simulink model "nav"  (R2025b)
settings: Solver=ode2  StartTime=0.0  StopTime=inf  FixedStep=1/100  RelTol=1e-3
PreLoadFcn:
  | nav_PreLoadFcn
  | stepsize_ctrl = evalin('base', get_param(bdroot, 'FixedStep'));
values from neighbouring files (symbols this model uses):
  navConsts = defineConstants_nav()    [nav_PreLoadFcn.m]
undefined symbols (not defined in the file or in its folder): dspblkCoreblockFVToolHelper, gcbh
libraries: eeGeneralControl x5, simulink x2, sharedutil x1, sharedtransform x1
(part 1 of 2)
settings Model: Creator=ac112430  LastModifiedBy=ac124458
settings SolverCC: AlgebraicLoopSolver=TrustRegion
settings DataIOCC: ReturnWorkspaceOutputs=off
settings OptimizationCC: DefaultParameterBehavior=Inlined  DefaultUnderspecifiedDataType=single  PassReuseOutputArgsAs=Individual arguments  EfficientTunableParamExpr=on
settings DebuggingCC: ParameterPrecisionLossMsg=none  ParameterTunabilityLossMsg=error  UnconnectedInputMsg=warning  UnconnectedOutputMsg=warning  UnconnectedLineMsg=warning  BusObjectLabelMismatch=none  ArithmeticOperatorsInVariantConditions=warning
settings HardwareCC: ProdBitPerPointer=32.0  ProdBitPerSizeT=32.0  ProdBitPerPtrDiffT=32.0  ProdLargestAtomicInteger=Long  ProdLargestAtomicFloat=Double  ProdIntDivRoundTo=Undefined  ProdWordSize=32.0  ProdHWDeviceType=ARM Compatible->ARM Cortex
settings ModelReferenceCC: EnableRefExpFcnMdlSchedulingChecks=on  ModelReferenceNumInstancesAllowed=Single  PropagateSignalLabelsOutOfModel=off
settings SFSimCC: SimUseLocalCustomCode=off  MATLABDynamicMemAlloc=off  CustomCodeUndefinedFunction=UseInterfaceOnly
settings RTWCC: SystemTargetFile=ert.tlc  GenCodeOnly=on  TemplateMakefile=ert_default_tmf  RTWUseLocalCustomCode=off  IncludeHyperlinkInReport=on  GPUComputeCapability=3.5  Description=Embedded Coder
settings CodeAppCC: IgnoreCustomStorageClasses=off  MaxIdLength=2048.0  StateflowObjectComments=on
settings ERTTargetCC: ERTCustomFileTemplate=example_file_process.tlc  ConvertIfToSwitch=off  SuppressUnreachableDefaultCases=off  DynamicArrayContainerType=coder::array  TargetLangStandard=C99 (ISO)  GenerateSampleERTMain=on  SubcomponentCodeInterfacePackaging=Nonreusable function  SupportNonFinite=off  SupportComplex=off

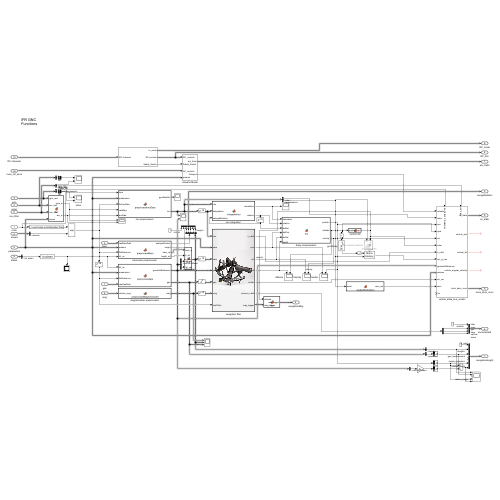
[thumbnail: Simulink's stored preview of the top-level diagram]
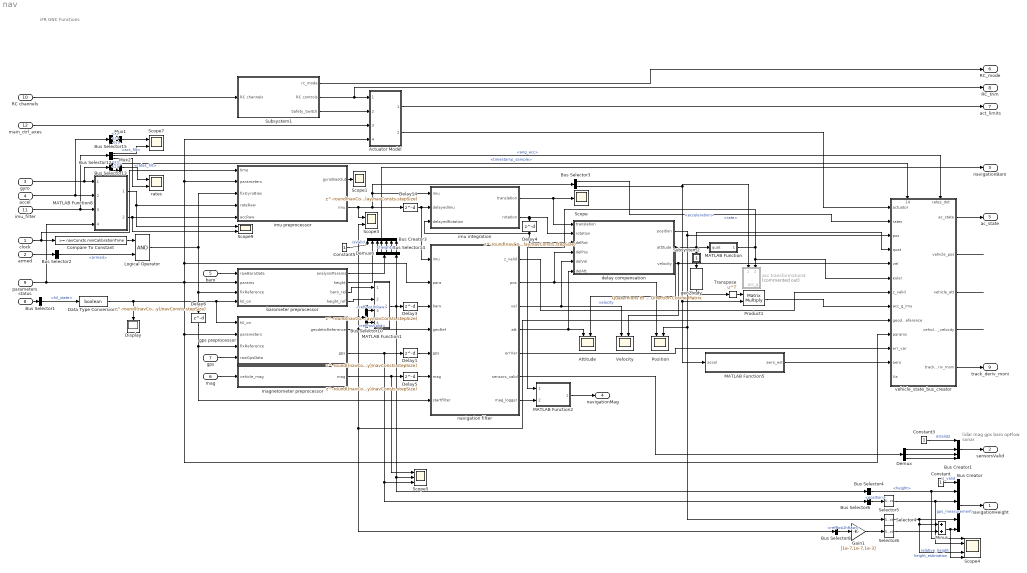
== system nav ==
  note: lidar
      | mag
      | gps
      | baro
      | opFlow
      | sonar
  note: iFR GNC Functions
  clock : Inport  OutDataTypeStr=single
  armed : Inport  Port=2  OutDataTypeStr=Bus: actuator_armed_bus
  gyro : Inport  Port=3  OutDataTypeStr=Bus: sensor_gyro_bus
  accel : Inport  Port=4  OutDataTypeStr=Bus: sensor_accel_bus
  baro : Inport  Port=5  OutDataTypeStr=Bus: sensor_baro_bus
  mag : Inport  Port=6  OutDataTypeStr=Bus: vehicle_magnetometer_bus
  gps : Inport  Port=7  OutDataTypeStr=Bus: vehicle_gps_position_bus
  status : Inport  Port=8  OutDataTypeStr=Bus: vehicle_status_bus  Interpolate=off  BusOutputAsStruct=on
  parameters : Inport  Port=9  OutDataTypeStr=Bus: nav_parameterBus
  RC channels : Inport  Port=10  OutDataTypeStr=Bus: rc_channels_bus
  imu_filter : Inport  Port=11  OutDataTypeStr=Bus: ifr_imu_filtered_bus
  main_ctrl_axes : Inport  Port=12  OutDataTypeStr=Bus: main_ctrl_axes_bus
  Actuator Model : Subsystem
  Attitude : Scope  NumInputPorts=2
      settings: ActiveDisplayYMinimum=-1.23773  ActiveDisplayYMaximum=1.24864
  Bus Creator : BusCreator  Inputs=6
  Bus Creator1 : BusCreator  Inputs=5
  Bus Creator3 : BusCreator  Inputs=7
  Bus Selector1 : BusSelector  OutputSignals=hil_state
  Bus Selector10 : BusSelector  OutputSignals=refPosLlhRaw,refPosValid
  Bus Selector12 : BusSelector  OutputSignals=acc_filt,ang_acc,rates_filt
  Bus Selector13 : BusSelector  OutputSignals=timestamp_sample,x,y,z
  Bus Selector14 : BusSelector  OutputSignals=height
  Bus Selector15 : BusSelector  OutputSignals=x,y,z
  Bus Selector2 : BusSelector  OutputSignals=armed
  Bus Selector3 : BusSelector  OutputSignals=rate,acceleration
  Bus Selector4 : BusSelector  OutputSignals=height
  Bus Selector6 : BusSelector  OutputSignals=position
  Bus Selector8 : BusSelector  OutputSignals=refPosLlhRaw
  Compare To Constant : simulink/Logic and Bit Operations/Compare To Constant  relop=>=  const=navConsts.minCalibrationTime  OutDataTypeStr=boolean
  Constant : Constant  OutDataTypeStr=boolean
  Constant3 : Constant  OutDataTypeStr=boolean
  Constant5 : Constant  OutDataTypeStr=boolean
  Data Type Conversion1 : DataTypeConversion  OutDataTypeStr=boolean  SaturateOnIntegerOverflow=off  RndMeth=Floor
  Delay1 : Delay  DelayLength=round((navConsts.filterDelay-navConsts.gpsDelay)/navConsts.stepSize)  DelayLengthUpperLimit=300
  Delay14 : Delay  DelayLength=round(navConsts.filterDelay/navConsts.stepSize)  DelayLengthUpperLimit=300
  Delay3 : Delay  DelayLength=round(navConsts.filterDelay/navConsts.stepSize)  DelayLengthUpperLimit=300
  Delay4 : Delay  DelayLength=round(navConsts.filterDelay/navConsts.stepSize)  DelayLengthUpperLimit=300
  Delay5 : Delay  DelayLength=round((navConsts.filterDelay-navConsts.magDelay)/navConsts.stepSize)  DelayLengthUpperLimit=300
  Delay6 : Delay  DelayLength=round((navConsts.filterDelay-navConsts.magDelay)/navConsts.stepSize)  DelayLengthUpperLimit=300
  Demux : Demux  Outputs=3
  Demux6 : Demux
  Display : Display
  Gain1 : Gain  Gain=[1e-7,1e-7,1e-3]  OutDataTypeStr=single
  Logical Operator : Logic  AllPortsSameDT=off  OutDataTypeStr=boolean
  MATLAB Function : MATLAB Function  TreatAsAtomicUnit=on
  MATLAB Function1 : MATLAB Function  TreatAsAtomicUnit=on
  MATLAB Function2 : MATLAB Function  TreatAsAtomicUnit=on
  MATLAB Function5 : MATLAB Function  TreatAsAtomicUnit=on
  MATLAB Function8 : MATLAB Function  TreatAsAtomicUnit=on
  Minus : Sum  OutDataTypeStr=single
  Mux1 : Mux  Inputs=3
  Mux2 : Mux  Inputs=3
  Position : Scope  NumInputPorts=2
      settings: ActiveDisplayYMinimum=-398.4041  ActiveDisplayYMaximum=44.26944  DataLoggingVariableName=ScopeData2
  Product1 : Product  Multiplication=Matrix(*)
  Scope : Scope
      settings: ActiveDisplayYMinimum=-1  ActiveDisplayYMaximum=1  DataLoggingVariableName=ScopeData5
  Scope1 : Scope
      settings: ActiveDisplayYMinimum=-0.099331239782016356  ActiveDisplayYMaximum=0.30195901907356948  DataLoggingVariableName=ScopeData4
  Scope3 : Scope  NumInputPorts=2
      settings: ActiveDisplayYMinimum=-0.2713911799557156  ActiveDisplayYMaximum=0.36740796754492377
  Scope4 : Scope  NumInputPorts=5
      settings: ActiveDisplayYMinimum=349.247314453125  ActiveDisplayYMaximum=356.774169921875
  Scope5 : Scope  NumInputPorts=3
      settings: ActiveDisplayYMinimum=349.247314453125  ActiveDisplayYMaximum=356.774169921875  DataLoggingVariableName=ScopeData2
  Scope7 : Scope  NumInputPorts=2
      settings: ActiveDisplayYMinimum=-34.351112127304077  ActiveDisplayYMaximum=34.884191274642944  DataLoggingVariableName=ScopeData10
  Scope9 : Scope  NumInputPorts=2
      settings: ActiveDisplayYMinimum=-1.8034829497337341  ActiveDisplayYMaximum=1.8379871249198914  DataLoggingVariableName=ScopeData13
  Selector4 : Selector  InputPortWidth=3  IndexOptions=Index vector (dialog)  Indices=[3]  OutputSizes=1
  Selector5 : Selector  InputPortWidth=3  IndexOptions=Index vector (dialog)  Indices=[3]  OutputSizes=1
  Selector6 : Selector  InputPortWidth=3  IndexOptions=Index vector (dialog)  Indices=[3]  OutputSizes=1
  Subsystem1 : Subsystem
  Subsystem2 : Subsystem
  Transpose : Math  Operator=transpose  SignedPower=on
  Velocity : Scope  NumInputPorts=2
      settings: ActiveDisplayYMinimum=-1  ActiveDisplayYMaximum=1  DataLoggingVariableName=ScopeData6
  acc transformation4 : MATLAB Function  Commented=on  TreatAsAtomicUnit=on
  barometer preprocessor : MATLAB Function  TreatAsAtomicUnit=on
  delay compensation : MATLAB Function  TreatAsAtomicUnit=on
  geo2body : sharedtransform/Quaternions to  Direction Cosine Matrix  aMode=aMode
  gps preprocessor : MATLAB Function  TreatAsAtomicUnit=on
  imu integration : MATLAB Function  TreatAsAtomicUnit=on
  imu preprocessor : MATLAB Function  TreatAsAtomicUnit=on
  magnetometer preprocessor : MATLAB Function  TreatAsAtomicUnit=on
  navigation filter : MATLAB Function  TreatAsAtomicUnit=on
  rates : Scope  NumInputPorts=2
      settings: ActiveDisplayYMinimum=-0.071955539506195931  ActiveDisplayYMaximum=0.11984543374486778  DataLoggingVariableName=ScopeData12
  vehicle_state_bus_creator : Subsystem
      settings: PortSchema="{\"entries\":[{\"content\":{\"sides\":[{\"content\":{\"connectorIds\":[\"In1\",\"In2\",\"In3\",\"In4\",\"In5\",\"In6\",\"In7\",\"In8\",\"In9\",\"In10\",\"In11\",\"In12\",\"In13\"]},\"type\":\"ConnectorPlacement.EquallySpacedRectSide\",\"uuid\":\"bc3ebfa1-daea-4709-952f-2fe4ea6771b8\"},{\"content\":{\"connectorIds\":[\"Out1\",\"Out2\",\"Out3\",\"Out4\",\"Out5\"],\"side\":\"RIGHT\"},\"type\":\"ConnectorPlacement.EquallySpacedRectSide\",\"uuid\":\"b99c6143-0656-4628-8455-051c6ced2792\"},{\"content\":{\"connectorIds\":[\"In14\",\"In15\"],\"side\":\"TOP\"},\"type\":\"ConnectorPlacement.EquallySpacedRectSide\",\"uuid\":\"81670970-0de5-4bc9-ac84-25aad24a7ec1\"},{\"content\":{\"side\":\"BOTTOM\"},\"type\":\"ConnectorPlacement.EquallySpacedRectSide\",\"uuid\":\"a3441f3b-1f80-4af6-b92c-bd0c79ef418a\"}]},\"type\":\"ConnectorPlacement.EquallySpacedConnector\",\"uuid\":\"3c725a23-f94b-421e-875e-8459dec9d453\"}],\"packageUris\":[\"http://schema.mathworks.com/mf0/Connector/R2020b\"],\"version\":\"1.0\"}"
  navigationHeight : Outport  OutDataTypeStr=Bus: navigation_height_bus
  sensorsValid : Outport  Port=2  OutDataTypeStr=Bus: sensors_valid_bus  VectorParamsAs1DForOutWhenUnconnected=off
  navigationBaro : Outport  Port=3  OutDataTypeStr=Bus: navigation_baro_bus  VectorParamsAs1DForOutWhenUnconnected=off
  navigationMag : Outport  Port=4  OutDataTypeStr=Bus: navigation_mag_bus
  ac_state : Outport  Port=5  OutDataTypeStr=Bus: vehicle_state_bus  VectorParamsAs1DForOutWhenUnconnected=off
  RC_mode : Outport  Port=6  OutDataTypeStr=Bus: rc_mode_bus
  act_limits : Outport  Port=7  OutDataTypeStr=Bus: actuator_limits_bus
  RC_trim : Outport  Port=8  OutDataTypeStr=Bus: rc_trim_bus
  track_deriv_moni : Outport  Port=9  OutDataTypeStr=Bus: track_deriv_monitor_bus
  wires:
  MATLAB Function8/1(gyro_m) -> Scope9/1, imu preprocessor/4(rateRaw)
  Demux/1 -> Bus Creator1/3
  baro/1 -> barometer preprocessor/1(rawBaroData)
  imu integration/2(rotation) -> delay compensation/2(rotation), Delay4/1
  Bus Selector6/1 -> Selector5/1  "<position>"
  Selector5/1 -> Scope4/2, Bus Creator/3  "gps_measurement"
  Selector4/1 -> Bus Creator/5, Scope4/4, Minus/1  "height_estimation"
  Bus Creator1/1 -> sensorsValid/1
  status/1 -> Bus Selector1/1
  Compare To Constant/1 -> Logical Operator/1
  Delay14/1 -> imu integration/2(delayedImu), navigation filter/1(imu)
  Bus Selector3/2 -> acc transformation4/1(acc_b), MATLAB Function5/1(accel), Product1/2  "<acceleration>"
  barometer preprocessor/2(height) -> Bus Creator3/2
  gps preprocessor/2(gps) -> Delay1/1, Scope5/3, Bus Selector6/1
  Bus Selector3/1 -> vehicle_state_bus_creator/2(rates)  "<rate>"
  navigation filter/3(vel) -> Velocity/1, delay compensation/5(delVel)  "velocity"
  Bus Selector1/1 -> Data Type Conversion1/1  "<hil_state>"
  barometer preprocessor/3(baro_rel) -> MATLAB Function1/1(baro_rel)
  navigation filter/6(sensors_valid) -> Demux/1
  delay compensation/1(position) -> vehicle_state_bus_creator/3(pos), Selector4/1, Position/2
  Bus Selector2/1 -> Logical Operator/2  "<armed>"
  Delay3/1 -> navigation filter/3(baro)
  magnetometer preprocessor/1(mag) -> Scope5/1, Delay5/1
  imu preprocessor/1(gyroBiasOut) -> Scope1/1
  Demux/2 -> Bus Creator1/4
  Demux6/2 -> Bus Creator3/4
  Constant/1 -> Bus Creator/1  "is_valid"
  Delay5/1 -> navigation filter/6(mag)
  Bus Creator3/1 -> navigationBaro/1
  armed/1 -> Bus Selector2/1
  Demux/3 -> Bus Creator1/5
  Constant3/1 -> Bus Creator1/1  "isValid2"
  clock/1 -> imu preprocessor/1(time), Compare To Constant/1
  Transpose/1 -> Product1/1
  Logical Operator/1 -> Delay6/1, barometer preprocessor/3(fixReference), imu preprocessor/3(fixGyroBias)
  Delay4/1 -> delay compensation/3(delRot), imu integration/3(delayedRotation)
  Bus Creator/1 -> navigationHeight/1
  geo2body/1 -> Transpose/1
  Bus Selector4/1 -> Bus Creator/2, Scope4/1  "<height>"
  navigation filter/2(pos) -> Position/1, delay compensation/4(delPos)
  imu preprocessor/2(imu) -> Bus Selector3/1, imu integration/1(imu), Delay14/1, Scope3/1
  Constant5/1 -> Bus Creator3/1  "isValid"
  Demux6/1 -> Bus Creator3/3
  Product1/1 -> vehicle_state_bus_creator/8(acc_g_imu)
  Delay1/1 -> navigation filter/5(gps)
  Data Type Conversion1/1 -> gps preprocessor/1(hil_on), barometer preprocessor/4(hil_on), Display/1
  imu integration/1(translation) -> Scope/1, delay compensation/1(translation)
  mag/1 -> magnetometer preprocessor/1(vehicle_mag)
  navigation filter/4(att) -> delay compensation/6(delAtt), Attitude/1
  MATLAB Function/1(eul_rad) -> vehicle_state_bus_creator/6(euler), acc transformation4/2(euler), MATLAB Function2/1(attitude)
  barometer preprocessor/1(analysisParams) -> Demux6/1
  Demux6/3 -> Bus Creator3/5
  Minus/1 -> Scope4/5, Bus Creator/6  "relative_height"
  MATLAB Function1/1(baro_abs) -> Bus Selector14/1, Scope5/2, Bus Selector4/1, Delay3/1
  Bus Selector10/1 -> MATLAB Function1/3(ref_pos)  "<refPosLlhRaw>"
  barometer preprocessor/4(height_ref) -> MATLAB Function1/2(h_ref)
  Demux6/4 -> Bus Creator3/6
  gps preprocessor/1(geodeticReference) -> Scope3/2, Bus Selector10/1, vehicle_state_bus_creator/9(geodeticReference), Bus Selector8/1, navigation filter/4(geoRef)
  Bus Selector10/2 -> MATLAB Function1/4(ref_valid)  "<refPosValid>"
  navigation filter/7(mag_logger) -> MATLAB Function2/2("mag_logger ")
  MATLAB Function2/1(mag_logger) -> navigationMag/1
  MATLAB Function8/2(acc_m) -> imu preprocessor/5(accRaw), Scope9/2
  MATLAB Function5/1(aero_est) -> vehicle_state_bus_creator/12(aero)
  delay compensation/3(velocity) -> vehicle_state_bus_creator/5(vel), Velocity/2
  parameters/1 -> MATLAB Function8/4(param), Actuator Model/4(params), imu preprocessor/2(parameters), navigation filter/2(para), barometer preprocessor/2(params), vehicle_state_bus_creator/10(params), gps preprocessor/2(parameters)
  main_ctrl_axes/1 -> Actuator Model/3(AP_controls)
  Subsystem1/3(Safety_Switch) -> Actuator Model/2(Safety_Switch)
  Actuator Model/2(Delayed) -> vehicle_state_bus_creator/1(actuator)
  RC channels/1 -> Subsystem1/1(RC channels)
  Subsystem1/1(rc_mode) -> RC_mode/1
  vehicle_state_bus_creator/1(ac_state) -> ac_state/1
  navigation filter/5(errVar) -> vehicle_state_bus_creator/11(err_var)
  navigation filter/1(z_valid) -> vehicle_state_bus_creator/7(z_valid)
  Gain1/1 -> Selector6/1
  Selector6/1 -> Minus/2
  Actuator Model/1(act_limits) -> act_limits/1
  Subsystem1/2(RC controls) -> RC_trim/1, Actuator Model/1(RC_controls)
  gps/1 -> gps preprocessor/4(rawGpsData)
  Delay6/1 -> gps preprocessor/3(fixReference), navigation filter/7(startFilter)
  delay compensation/2(attitude) -> vehicle_state_bus_creator/4(quat), MATLAB Function/1(quat), Subsystem2/1(" "), Attitude/2
  Subsystem2/1(Out1) -> geo2body/1
  Bus Selector8/1 -> Gain1/1  "<refPosLlhRaw>"
  vehicle_state_bus_creator/3(vehicle_att) -> ?
  vehicle_state_bus_creator/2(vehicle_pos) -> ?
  Bus Selector13/1 -> vehicle_state_bus_creator/14(timestamp_sample_imu)  "<timestamp_sample>"
  vehicle_state_bus_creator/5(track_deriv_moni) -> track_deriv_moni/1
  imu_filter/1 -> Bus Selector12/1, MATLAB Function8/3(imu_filter)
  accel/1 -> Bus Selector15/1, MATLAB Function8/2(acc_raw)
  gyro/1 -> Bus Selector13/1, MATLAB Function8/1(gyro_raw)
  Bus Selector12/2 -> vehicle_state_bus_creator/15(rates_dot)  "<ang_acc>"
  Bus Selector14/1 -> Bus Creator3/7  "<height>"
  Bus Selector15/1 -> Mux1/1  "<x>"
  Bus Selector15/2 -> Mux1/2  "<y>"
  Bus Selector15/3 -> Mux1/3  "<z>"
  Mux1/1 -> Scope7/1
  Bus Selector13/2 -> Mux2/1  "<x>"
  Bus Selector13/3 -> Mux2/2  "<y>"
  Bus Selector13/4 -> Mux2/3  "<z>"
  Mux2/1 -> rates/1
  Bus Selector12/1 -> Scope7/2  "<acc_filt>"
  Bus Selector12/3 -> rates/2  "<rates_filt>"
  vehicle_state_bus_creator/4(vehicle_angular_velocity) -> ?

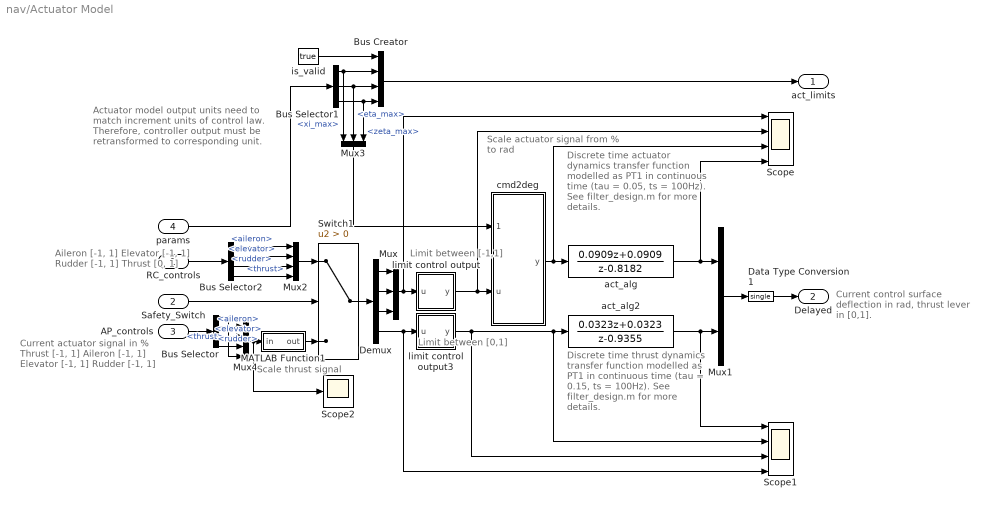
== system nav/Actuator Model ==
  note: Discrete time actuator
      | dynamics transfer function
      | modelled as PT1 in
      | continuous time (tau = 0.05,
      | ts = 100Hz).
      | See filter_design.m for
      | more details.
  note: Actuator model output units need to
      | match increment units of control law.
      | Therefore, controller output must be
      | retransformed to corresponding unit.
  note: Current control surface
      | deflection in rad, thrust
      | lever in [0,1].
  note: Current actuator signal in %
      | Thrust [-1, 1]
      | Aileron [-1, 1]
      | Elevator [-1, 1]
      | Rudder [-1, 1]
  note: Scale actuator
      | signal from
      | % to rad
  note: Limit between
      | [-1,1]
  note: Limit
      | between
      | [0,1]
  note: Discrete time thrust
      | dynamics transfer function
      | modelled as PT1 in
      | continuous time (tau = 0.15,
      | ts = 100Hz).
      | See filter_design.m for
      | more details.
  note: Aileron		[-1, 1]
      | Elevator		[-1, 1]
      | Rudder		[-1, 1]
      | Thrust		[0, 1]
  note: Scale thrust signal
  RC_controls : Inport  OutDataTypeStr=Bus: rc_trim_bus
  Safety_Switch : Inport  Port=2
  AP_controls : Inport  Port=3  OutDataTypeStr=Bus: main_ctrl_axes_bus
  params : Inport  Port=4  OutDataTypeStr=Bus: nav_parameterBus
  Bus Creator : BusCreator  Inputs=4  OutDataTypeStr=Bus: actuator_limits_bus
      settings: InheritFromInputs=off
  Bus Selector : BusSelector  OutputSignals=thrust,aileron,elevator,rudder
  Bus Selector1 : BusSelector  OutputSignals=xi_max,eta_max,zeta_max
  Bus Selector2 : BusSelector  OutputSignals=aileron,elevator,rudder,thrust
  Data Type Conversion1 : DataTypeConversion  OutDataTypeStr=single  SaturateOnIntegerOverflow=off  RndMeth=Floor
  Demux : Demux
  MATLAB Function1 : MATLAB Function  TreatAsAtomicUnit=on
  Mux : Mux  Inputs=3
  Mux1 : Mux  Inputs=2
  Mux2 : Mux
  Mux3 : Mux  Inputs=3
  Mux4 : Mux
  Scope : Scope  NumInputPorts=4
  Scope1 : Scope  NumInputPorts=4
      settings: ActiveDisplayYMinimum=-0.125  ActiveDisplayYMaximum=1.125
  Scope2 : Scope
      settings: ActiveDisplayYMinimum=-1  ActiveDisplayYMaximum=1  DataLoggingVariableName=ScopeData8
  Switch1 : Switch  Criteria=u2 > Threshold  SaturateOnIntegerOverflow=off  InputSameDT=off
  act_alg : DiscreteTransferFcn  Numerator=[0.0909 0.0909]  Denominator=[1 -0.8182]
  act_alg2 : DiscreteTransferFcn  LoadFcn=dspblkCoreblockFVToolHelper(gcbh,'load');  Numerator=[0.0323 0.0323]  Denominator=[1 -0.9355]
      settings: CopyFcn=dspblkCoreblockFVToolHelper(gcbh,'copy');  DeleteFcn=dspblkCoreblockFVToolHelper(gcbh,'close');  ModelCloseFcn=dspblkCoreblockFVToolHelper(gcbh,'close');  PreSaveFcn=dspblkCoreblockFVToolHelper(gcbh,'presave');  PostSaveFcn=dspblkCoreblockFVToolHelper(gcbh,'postsave');  CloseFcn=dspblkCoreblockFVToolHelper(gcbh,'close');
  cmd2deg : MATLAB Function  TreatAsAtomicUnit=on
  is_valid : Constant  Value=true
  limit control output : MATLAB Function  TreatAsAtomicUnit=on
  limit control output3 : MATLAB Function  TreatAsAtomicUnit=on
  act_limits : Outport  OutDataTypeStr=Bus: actuator_limits_bus
  Delayed : Outport  Port=2
  wires:
  act_alg2/1 -> Scope1/1, Mux1/2
  limit control output3/1(y) -> Scope1/2, act_alg2/1, Scope1/3
  params/1 -> Bus Selector1/1
  Mux1/1 -> Data Type Conversion1/1
  act_alg/1 -> Scope/4, Mux1/1
  Demux/3 -> Mux/3
  Demux/1 -> Mux/1
  Demux/2 -> Mux/2
  AP_controls/1 -> Bus Selector/1
  Data Type Conversion1/1 -> Delayed/1
  Mux4/1 -> Scope2/1, MATLAB Function1/1(in)
  Mux/1 -> Scope/1, limit control output/1(u)
  cmd2deg/1(y) -> Scope/3, act_alg/1
  limit control output/1(y) -> Scope/2, cmd2deg/2(u)
  RC_controls/1 -> Bus Selector2/1
  MATLAB Function1/1(out) -> Switch1/3
  Bus Selector/1 -> Mux4/4  "<thrust>"
  Bus Selector1/1 -> Bus Creator/2, Mux3/1  "<xi_max>"
  Bus Creator/1 -> act_limits/1
  is_valid/1 -> Bus Creator/1
  Demux/4 -> Scope1/4, limit control output3/1(u)
  Mux2/1 -> Switch1/1
  Bus Selector2/1 -> Mux2/1  "<aileron>"
  Bus Selector2/2 -> Mux2/2  "<elevator>"
  Bus Selector2/3 -> Mux2/3  "<rudder>"
  Bus Selector2/4 -> Mux2/4  "<thrust>"
  Bus Selector1/2 -> Mux3/2, Bus Creator/3  "<eta_max>"
  Bus Selector1/3 -> Mux3/3, Bus Creator/4  "<zeta_max>"
  Safety_Switch/1 -> Switch1/2
  Mux3/1 -> cmd2deg/1(act_limits)
  Switch1/1 -> Demux/1
  Bus Selector/2 -> Mux4/1  "<aileron>"
  Bus Selector/3 -> Mux4/2  "<elevator>"
  Bus Selector/4 -> Mux4/3  "<rudder>"

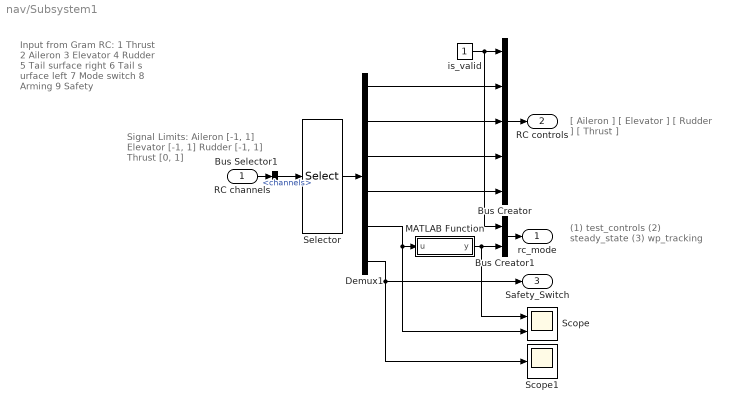
== system nav/Subsystem1 ==
  note: Input from Gram RC:
      | 1 Thrust
      | 2 Aileron
      | 3 Elevator
      | 4 Rudder
      | 5 Tail surface right
      | 6 Tail s urface left
      | 7 Mode switch
      | 8 Arming
      | 9 Safety
  note: Signal Limits:
      | Aileron		[-1, 1]
      | Elevator		[-1, 1]
      | Rudder		[-1, 1]
      | Thrust		[0, 1]
  note: (1) test_controls
      | (2) steady_state
      | (3) wp_tracking
  note: [ Aileron	  ]
      | [ Elevator ]
      | [ Rudder	  ]
      | [ Thrust	  ]
  RC channels : Inport  OutDataTypeStr=Bus: rc_channels_bus
  Bus Creator : BusCreator  Inputs=5  OutDataTypeStr=Bus: rc_trim_bus
      settings: InheritFromInputs=off
  Bus Creator1 : BusCreator  Inputs=2  OutDataTypeStr=Bus: rc_mode_bus
      settings: InheritFromInputs=off
  Bus Selector1 : BusSelector  OutputSignals=channels
  Demux1 : Demux  Outputs=6
  MATLAB Function : MATLAB Function  TreatAsAtomicUnit=on
  Scope : Scope  NumInputPorts=2
      settings: ActiveDisplayYMinimum=-1.5  ActiveDisplayYMaximum=3.5  DataLoggingVariableName=ScopeData3
  Scope1 : Scope
      settings: ActiveDisplayYMinimum=-1.5  ActiveDisplayYMaximum=3.5  DataLoggingVariableName=ScopeData7
  Selector : Selector  InputPortWidth=18  IndexOptions=Index vector (dialog)  Indices=[2 3 4 1 7 9]  OutputSizes=1
  is_valid : Constant  OutDataTypeStr=boolean
  rc_mode : Outport  OutDataTypeStr=Bus: rc_mode_bus
  RC controls : Outport  Port=2  OutDataTypeStr=Bus: rc_trim_bus
  Safety_Switch : Outport  Port=3
  wires:
  Bus Creator/1 -> RC controls/1
  Demux1/1 -> Bus Creator/2
  Demux1/6 -> Safety_Switch/1, Scope1/1
  MATLAB Function/1(y) -> Bus Creator1/2, Scope/1
  Demux1/5 -> Scope/2, MATLAB Function/1(u)
  Selector/1 -> Demux1/1
  Demux1/3 -> Bus Creator/4
  RC channels/1 -> Bus Selector1/1
  Demux1/4 -> Bus Creator/5
  Bus Selector1/1 -> Selector/1  "<channels>"
  Demux1/2 -> Bus Creator/3
  Bus Creator1/1 -> rc_mode/1
  is_valid/1 -> Bus Creator1/1, Bus Creator/1

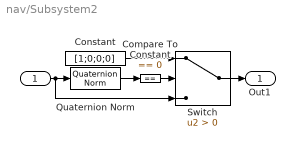
== system nav/Subsystem2 ==
  " " : Inport
  Compare To Constant : simulink/Logic and Bit Operations/Compare To Constant  relop===  const=0  OutDataTypeStr=boolean
  Constant : Constant  Value=[1;0;0;0]  OutDataTypeStr=single
  Quaternion Norm : sharedutil/Quaternion Norm  aMode=aMode
      settings: LibrarySourceBlock=|
      | aerolibutil/Quaternion
      | Norm
  Switch : Switch  Criteria=u2 > Threshold  SaturateOnIntegerOverflow=off  InputSameDT=off
  Out1 : Outport
  wires:
  " "/1 -> Switch/3, Quaternion Norm/1
  Quaternion Norm/1 -> Compare To Constant/1
  Compare To Constant/1 -> Switch/2
  Constant/1 -> Switch/1
  Switch/1 -> Out1/1

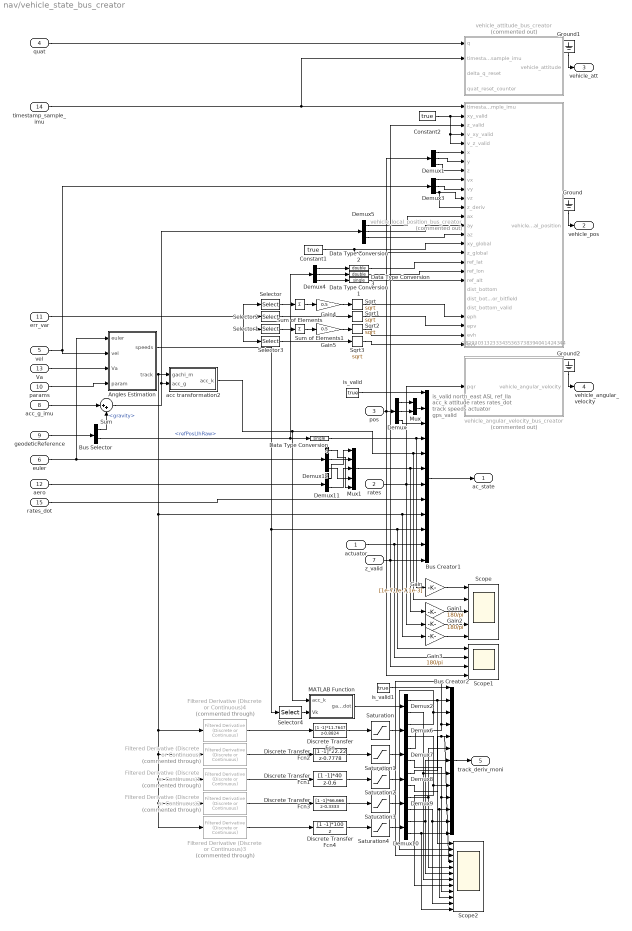
== system nav/vehicle_state_bus_creator ==
  note: is_valid
      |
      | north_east
      |
      | ASL
      |
      | ref_lla
      |
      | acc_k
      |
      | attitude
      |
      | rates
      |
      | rates_dot
      |
      | track
      |
      | speeds
      |
      | actuator
      |
      | gps_valid
  actuator : Inport
  rates : Inport  Port=2
  pos : Inport  Port=3  OutDataTypeStr=single  PortDimensions=3
  quat : Inport  Port=4
  vel : Inport  Port=5
  euler : Inport  Port=6
  z_valid : Inport  Port=7  OutDataTypeStr=boolean
  acc_g_imu : Inport  Port=8
  geodeticReference : Inport  Port=9  OutDataTypeStr=Bus: ifr_geodeticReference
  params : Inport  Port=10
  err_var : Inport  Port=11
  aero : Inport  Port=12
  Va : Inport  Port=13
  timestamp_sample_imu : Inport  Port=14
  rates_dot : Inport  Port=15
  Angles Estimation : MATLAB Function  TreatAsAtomicUnit=on
  Bus Selector : BusSelector  OutputSignals=gravity,refPosLlhRaw
  Bus Creator1 : BusCreator  Inputs=12  OutDataTypeStr=Bus: vehicle_state_bus
      settings: InheritFromInputs=off
  Bus Creator2 : BusCreator  Inputs=13  OutDataTypeStr=Bus: track_deriv_monitor_bus
      settings: InheritFromInputs=off
  Constant1 : Constant  Value=true  OutDataTypeStr=boolean
  Constant2 : Constant  Value=true  OutDataTypeStr=boolean
  Data Type Conversion1 : DataTypeConversion  OutDataTypeStr=double  SaturateOnIntegerOverflow=off  RndMeth=Floor
  Data Type Conversion2 : DataTypeConversion  OutDataTypeStr=double  SaturateOnIntegerOverflow=off  RndMeth=Floor
  Data Type Conversion3 : DataTypeConversion  OutDataTypeStr=single  SaturateOnIntegerOverflow=off  RndMeth=Floor
  Data Type Conversion4 : DataTypeConversion  OutDataTypeStr=single  SaturateOnIntegerOverflow=off  RndMeth=Floor
  Demux{,1,3..5,12} (6 alike) : Demux  Outputs=3
  Demux{2,6..11} (7 alike) : Demux  Outputs=2
  Discrete Transfer Fcn : DiscreteTransferFcn  LoadFcn=dspblkCoreblockFVToolHelper(gcbh,'load');  Numerator=[1 -1]*11.7647  Denominator=[1 -0.8824]
      settings: CopyFcn=dspblkCoreblockFVToolHelper(gcbh,'copy');  DeleteFcn=dspblkCoreblockFVToolHelper(gcbh,'close');  ModelCloseFcn=dspblkCoreblockFVToolHelper(gcbh,'close');  PreSaveFcn=dspblkCoreblockFVToolHelper(gcbh,'presave');  PostSaveFcn=dspblkCoreblockFVToolHelper(gcbh,'postsave');  CloseFcn=dspblkCoreblockFVToolHelper(gcbh,'close');
  Discrete Transfer Fcn1 : DiscreteTransferFcn  LoadFcn=dspblkCoreblockFVToolHelper(gcbh,'load');  Numerator=[1 -1]*40  Denominator=[1 -0.6]
      settings: CopyFcn=dspblkCoreblockFVToolHelper(gcbh,'copy');  DeleteFcn=dspblkCoreblockFVToolHelper(gcbh,'close');  ModelCloseFcn=dspblkCoreblockFVToolHelper(gcbh,'close');  PreSaveFcn=dspblkCoreblockFVToolHelper(gcbh,'presave');  PostSaveFcn=dspblkCoreblockFVToolHelper(gcbh,'postsave');  CloseFcn=dspblkCoreblockFVToolHelper(gcbh,'close');
  Discrete Transfer Fcn2 : DiscreteTransferFcn  LoadFcn=dspblkCoreblockFVToolHelper(gcbh,'load');  Numerator=[1 -1]*22.22  Denominator=[1 -0.7778]
      settings: CopyFcn=dspblkCoreblockFVToolHelper(gcbh,'copy');  DeleteFcn=dspblkCoreblockFVToolHelper(gcbh,'close');  ModelCloseFcn=dspblkCoreblockFVToolHelper(gcbh,'close');  PreSaveFcn=dspblkCoreblockFVToolHelper(gcbh,'presave');  PostSaveFcn=dspblkCoreblockFVToolHelper(gcbh,'postsave');  CloseFcn=dspblkCoreblockFVToolHelper(gcbh,'close');
  Discrete Transfer Fcn3 : DiscreteTransferFcn  LoadFcn=dspblkCoreblockFVToolHelper(gcbh,'load');  Numerator=[1 -1]*66.666  Denominator=[1 -0.3333]
      settings: CopyFcn=dspblkCoreblockFVToolHelper(gcbh,'copy');  DeleteFcn=dspblkCoreblockFVToolHelper(gcbh,'close');  ModelCloseFcn=dspblkCoreblockFVToolHelper(gcbh,'close');  PreSaveFcn=dspblkCoreblockFVToolHelper(gcbh,'presave');  PostSaveFcn=dspblkCoreblockFVToolHelper(gcbh,'postsave');  CloseFcn=dspblkCoreblockFVToolHelper(gcbh,'close');
  Discrete Transfer Fcn4 : DiscreteTransferFcn  LoadFcn=dspblkCoreblockFVToolHelper(gcbh,'load');  Numerator=[1 -1]*100  Denominator=[1 0]
      settings: CopyFcn=dspblkCoreblockFVToolHelper(gcbh,'copy');  DeleteFcn=dspblkCoreblockFVToolHelper(gcbh,'close');  ModelCloseFcn=dspblkCoreblockFVToolHelper(gcbh,'close');  PreSaveFcn=dspblkCoreblockFVToolHelper(gcbh,'presave');  PostSaveFcn=dspblkCoreblockFVToolHelper(gcbh,'postsave');  CloseFcn=dspblkCoreblockFVToolHelper(gcbh,'close');
  Filtered Derivative (Discrete or Continuous) : eeGeneralControl/Filtered Derivative (Discrete or Continuous)  Commented=through  K=1  T=0.04  B=inf  A=-inf  minRatio=10  init_option=Inherited from block input  x0=0  Ts=-1
      settings: LibrarySourceBlock=|
      | ee_sl_lib/General Control/Filtered Derivative
      | (Discrete or Continuous)
  Filtered Derivative (Discrete or Continuous)1 : eeGeneralControl/Filtered Derivative (Discrete or Continuous)  Commented=through  K=1  T=0.02  B=inf  A=-inf  minRatio=10  init_option=Inherited from block input  x0=0  Ts=-1
      settings: LibrarySourceBlock=|
      | ee_sl_lib/General Control/Filtered Derivative
      | (Discrete or Continuous)
  Filtered Derivative (Discrete or Continuous)2 : eeGeneralControl/Filtered Derivative (Discrete or Continuous)  Commented=through  K=1  T=0.01  B=inf  A=-inf  minRatio=10  init_option=Inherited from block input  x0=0  Ts=-1
      settings: LibrarySourceBlock=|
      | ee_sl_lib/General Control/Filtered Derivative
      | (Discrete or Continuous)
  Filtered Derivative (Discrete or Continuous)3 : eeGeneralControl/Filtered Derivative (Discrete or Continuous)  Commented=through  K=1  T=0.005  B=inf  A=-inf  minRatio=10  init_option=Inherited from block input  x0=0  Ts=-1
      settings: LibrarySourceBlock=|
      | ee_sl_lib/General Control/Filtered Derivative
      | (Discrete or Continuous)
  Filtered Derivative (Discrete or Continuous)4 : eeGeneralControl/Filtered Derivative (Discrete or Continuous)  Commented=through  K=1  T=0.08  B=inf  A=-inf  minRatio=10  init_option=Inherited from block input  x0=0  Ts=-1
      settings: LibrarySourceBlock=|
      | ee_sl_lib/General Control/Filtered Derivative
      | (Discrete or Continuous)
  Gain : Gain  Gain=[1e-7,1e-7,1e-3]
  Gain1 : Gain  Gain=180/pi
  Gain2 : Gain  Gain=180/pi
  Gain3 : Gain  Gain=180/pi
  Gain4 : Gain  Gain=0.5  OutDataTypeStr=single
  Gain5 : Gain  Gain=0.5  OutDataTypeStr=single
  Ground : Ground
  Ground1 : Ground
  Ground2 : Ground
  MATLAB Function : MATLAB Function  TreatAsAtomicUnit=on
  Mux : Mux  Inputs=2
  Mux1 : Mux  Inputs=5
  Saturation{,1..4} (5 alike) : Saturate  UpperLimit=pi  LowerLimit=-pi
  Scope : Scope  NumInputPorts=5
      settings: ActiveDisplayYMinimum=254.91900634765625  ActiveDisplayYMaximum=454.91900634765625
  Scope1 : Scope  NumInputPorts=4
      settings: ActiveDisplayYMinimum=-6.2473122477531415  ActiveDisplayYMaximum=73.263225734233856
  Scope2 : Scope  NumInputPorts=12
      settings: ActiveDisplayYMinimum=-3.0551776138868192  ActiveDisplayYMaximum=3.0376622643888282  DataLoggingVariableName=ScopeData9
  Selector : Selector  InputPortWidth=9  IndexOptions=Index vector (dialog)  Indices=[1 2]  OutputSizes=1
  Selector1 : Selector  InputPortWidth=9  IndexOptions=Index vector (dialog)  Indices=[4 5]  OutputSizes=1
  Selector2 : Selector  InputPortWidth=9  IndexOptions=Index vector (dialog)  Indices=3  OutputSizes=1
  Selector3 : Selector  InputPortWidth=9  IndexOptions=Index vector (dialog)  Indices=6  OutputSizes=1
  Selector4 : Selector  InputPortWidth=2  IndexOptions=Index vector (dialog)  Indices=1  OutputSizes=1
  Sqrt{,1..3} (4 alike) : Sqrt
  Sum : Sum  Inputs=|++
  Sum of Elements : Sum  Inputs=+
  Sum of Elements1 : Sum  Inputs=+
  acc transformation2 : MATLAB Function  TreatAsAtomicUnit=on
  is_valid : Constant  Value=true  OutDataTypeStr=boolean
  is_valid1 : Constant  Value=true  OutDataTypeStr=boolean
  vehicle_angular_velocity_bus_creator : Subsystem  Commented=on
  vehicle_attitude_bus_creator : Subsystem  Commented=on
  vehicle_local_position_bus_creator : Subsystem  Commented=on
      settings: PortSchema="{\"entries\":[{\"content\":{\"sides\":[{\"content\":{\"connectorIds\":[\"In1\",\"In2\",\"In3\",\"In4\",\"In5\",\"In6\",\"In7\",\"In8\",\"In9\",\"In10\",\"In11\",\"In12\",\"In13\",\"In14\",\"In15\",\"In16\",\"In17\",\"In18\",\"In19\",\"In20\",\"In21\",\"In22\",\"In23\",\"In24\",\"In25\",\"In26\",\"In27\"]},\"type\":\"ConnectorPlacement.EquallySpacedRectSide\",\"uuid\":\"d7b85d5c-5599-4e88-82f1-b7fab1ef21b9\"},{\"content\":{\"connectorIds\":[\"Out1\"],\"side\":\"RIGHT\"},\"type\":\"ConnectorPlacement.EquallySpacedRectSide\",\"uuid\":\"699d4796-c4a5-400d-ae7f-d0fe809a1d5f\"},{\"content\":{\"side\":\"TOP\"},\"type\":\"ConnectorPlacement.EquallySpacedRectSide\",\"uuid\":\"a5a49804-595b-4b61-9074-ba74b998a229\"},{\"content\":{\"connectorIds\":[\"In28\",\"In29\",\"In30\",\"In31\",\"In32\",\"In33\",\"In34\",\"In35\",\"In36\",\"In37\",\"In38\",\"In39\",\"In40\",\"In41\",\"In42\",\"In43\",\"In44\"],\"side\":\"BOTTOM\"},\"type\":\"ConnectorPlacement.EquallySpacedRectSide\",\"uuid\":\"117ce955-faca-4d28-9193-e1fd103a05b2\"}]},\"type\":\"ConnectorPlacement.EquallySpacedConnector\",\"uuid\":\"4d71e442-d8d4-4e8b-a7eb-573f45a4a9ae\"}],\"packageUris\":[\"http://schema.mathworks.com/mf0/Connector/R2020b\"],\"version\":\"1.0\"}"
  ac_state : Outport  OutDataTypeStr=Bus: vehicle_state_bus  VectorParamsAs1DForOutWhenUnconnected=off
  vehicle_pos : Outport  Port=2  OutDataTypeStr=Bus: vehicle_local_position_bus  VectorParamsAs1DForOutWhenUnconnected=off
  vehicle_att : Outport  Port=3  OutDataTypeStr=Bus: vehicle_attitude_bus  VectorParamsAs1DForOutWhenUnconnected=off
  vehicle_angular_velocity : Outport  Port=4  OutDataTypeStr=Bus: vehicle_angular_velocity_bus
  track_deriv_moni : Outport  Port=5  OutDataTypeStr=Bus: track_deriv_monitor_bus
  wires:
  is_valid/1 -> Bus Creator1/1
  euler/1 -> Angles Estimation/1(euler), Demux12/1
  aero/1 -> Demux11/1
  Demux11/2 -> Mux1/3
  Demux11/1 -> Mux1/1
  Demux12/3 -> Mux1/4
  Demux12/1 -> Mux1/5
  Demux12/2 -> Mux1/2
  actuator/1 -> Bus Creator1/11, Scope1/2
  rates/1 -> Gain2/1, vehicle_angular_velocity_bus_creator/1(pqr), Bus Creator1/7
  Angles Estimation/1(speeds) -> Selector4/1, Scope1/1, Bus Creator1/10
  Mux1/1 -> Gain1/1, Bus Creator1/6
  Mux/1 -> Bus Creator1/2
  Bus Creator1/1 -> ac_state/1
  Demux/3 -> Bus Creator1/3
  Demux/1 -> Mux/1
  Demux/2 -> Mux/2
  Gain/1 -> Scope/1
  Gain1/1 -> Scope/3
  Gain2/1 -> Scope/4
  Gain3/1 -> Scope/5
  z_valid/1 -> Bus Creator1/12, vehicle_local_position_bus_creator/3(z_valid), Scope1/3
  Constant2/1 -> vehicle_local_position_bus_creator/4(v_xy_valid), vehicle_local_position_bus_creator/5(v_z_valid), vehicle_local_position_bus_creator/2(xy_valid)
  Demux5/3 -> vehicle_local_position_bus_creator/15(az)
  Data Type Conversion1/1 -> vehicle_local_position_bus_creator/19(ref_lon)
  Sqrt3/1 -> vehicle_local_position_bus_creator/27(evv)
  acc transformation2/1(acc_k) -> MATLAB Function/1(acc_k), Scope/2, Bus Creator1/5
  Sqrt2/1 -> vehicle_local_position_bus_creator/26(evh)
  vel/1 -> Angles Estimation/2(vel), Demux3/1
  Demux4/3 -> Data Type Conversion3/1
  Sqrt1/1 -> vehicle_local_position_bus_creator/25(epv)
  Demux1/3 -> vehicle_local_position_bus_creator/8(z)
  Demux1/2 -> vehicle_local_position_bus_creator/7(y)
  Demux5/2 -> vehicle_local_position_bus_creator/14(ay)
  Constant1/1 -> vehicle_local_position_bus_creator/17(z_global), vehicle_local_position_bus_creator/16(xy_global)
  Demux1/1 -> vehicle_local_position_bus_creator/6(x)
  Data Type Conversion2/1 -> vehicle_local_position_bus_creator/18(ref_lat)
  Sqrt/1 -> vehicle_local_position_bus_creator/24(eph)
  Data Type Conversion3/1 -> vehicle_local_position_bus_creator/20(ref_alt)
  Demux3/3 -> vehicle_local_position_bus_creator/12(z_deriv), vehicle_local_position_bus_creator/11(vz)
  pos/1 -> Scope1/4, Demux1/1, Demux/1
  Demux5/1 -> vehicle_local_position_bus_creator/13(ax)
  Demux3/1 -> vehicle_local_position_bus_creator/9(vx)
  Demux3/2 -> vehicle_local_position_bus_creator/10(vy)
  Selector1/1 -> Sum of Elements1/1
  Selector/1 -> Sum of Elements/1
  Selector3/1 -> Sqrt3/1
  Sum of Elements1/1 -> Gain5/1
  Sum of Elements/1 -> Gain4/1
  Selector2/1 -> Sqrt1/1
  err_var/1 -> Selector/1, Selector1/1, Selector3/1, Selector2/1
  Gain5/1 -> Sqrt2/1
  Gain4/1 -> Sqrt/1
  Sum/1 -> Demux5/1, acc transformation2/2(acc_g)
  Bus Selector/2 -> Data Type Conversion4/1, Demux4/1  "<refPosLlhRaw>"
  Bus Selector/1 -> Sum/2  "<gravity>"
  geodeticReference/1 -> Bus Selector/1
  acc_g_imu/1 -> Sum/1
  Va/1 -> Angles Estimation/3(Va)
  params/1 -> Angles Estimation/4(param)
  Ground/1 -> vehicle_pos/1
  quat/1 -> vehicle_attitude_bus_creator/1(q)
  Ground1/1 -> vehicle_att/1
  timestamp_sample_imu/1 -> vehicle_attitude_bus_creator/2(timestamp_sample_imu), vehicle_local_position_bus_creator/1(timestamp_sample_imu)
  Demux4/2 -> Data Type Conversion1/1
  Demux4/1 -> Data Type Conversion2/1
  Data Type Conversion4/1 -> Gain/1, Bus Creator1/4
  MATLAB Function/1(gachi_dot) -> Demux2/1
  Filtered Derivative (Discrete or Continuous)4/1 -> Discrete Transfer Fcn/1
  Demux2/1 -> Bus Creator2/2, Scope2/1
  Demux6/1 -> Scope2/2, Bus Creator2/3
  Demux6/2 -> Scope2/8, Bus Creator2/9
  Demux2/2 -> Bus Creator2/8, Scope2/7
  is_valid1/1 -> Bus Creator2/1
  Bus Creator2/1 -> track_deriv_moni/1
  Selector4/1 -> MATLAB Function/2(Vk)
  Saturation/1 -> Demux6/1
  Filtered Derivative (Discrete or Continuous)/1 -> Discrete Transfer Fcn2/1
  Filtered Derivative (Discrete or Continuous)1/1 -> Discrete Transfer Fcn1/1
  Filtered Derivative (Discrete or Continuous)2/1 -> Discrete Transfer Fcn3/1
  Filtered Derivative (Discrete or Continuous)3/1 -> Discrete Transfer Fcn4/1
  Demux7/2 -> Scope2/9, Bus Creator2/10
  Demux8/2 -> Scope2/10, Bus Creator2/11
  Demux10/2 -> Scope2/12, Bus Creator2/13
  Saturation3/1 -> Demux9/1
  Saturation4/1 -> Demux10/1
  Saturation2/1 -> Demux8/1
  Saturation1/1 -> Demux7/1
  Demux9/2 -> Scope2/11, Bus Creator2/12
  Demux7/1 -> Scope2/3, Bus Creator2/4
  Demux8/1 -> Scope2/4, Bus Creator2/5
  Demux9/1 -> Bus Creator2/6, Scope2/5
  Demux10/1 -> Bus Creator2/7, Scope2/6
  rates_dot/1 -> Bus Creator1/8
  Angles Estimation/2(track) -> Gain3/1, Bus Creator1/9, Filtered Derivative (Discrete or Continuous)3/1, Filtered Derivative (Discrete or Continuous)2/1, Filtered Derivative (Discrete or Continuous)1/1, Filtered Derivative (Discrete or Continuous)/1, Filtered Derivative (Discrete or Continuous)4/1, acc transformation2/1(gachi_m)
  Discrete Transfer Fcn/1 -> Saturation/1
  Discrete Transfer Fcn2/1 -> Saturation1/1
  Discrete Transfer Fcn1/1 -> Saturation2/1
  Discrete Transfer Fcn3/1 -> Saturation3/1
  Discrete Transfer Fcn4/1 -> Saturation4/1
  Ground2/1 -> vehicle_angular_velocity/1

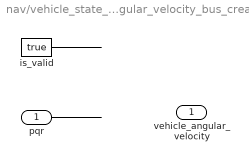
== system nav/vehicle_state_bus_creator/vehicle_angular_velocity_bus_creator ==
  pqr : Inport  OutDataTypeStr=single  PortDimensions=4
  is_valid : Constant  Value=true  OutDataTypeStr=boolean
  vehicle_angular_velocity : Outport  OutDataTypeStr=Bus: vehicle_angular_velocity_bus
  wires:
  ? -> ?
  ? -> ?
  pqr/1 -> ?
  ? -> ?
  is_valid/1 -> ?

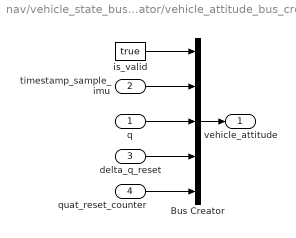
== system nav/vehicle_state_bus_creator/vehicle_attitude_bus_creator ==
  q : Inport  OutDataTypeStr=single  PortDimensions=4
  timestamp_sample_imu : Inport  Port=2
  delta_q_reset : Inport  Port=3  OutDataTypeStr=single  PortDimensions=4
  quat_reset_counter : Inport  Port=4  OutDataTypeStr=uint8  PortDimensions=1
  Bus Creator : BusCreator  Inputs=5  OutDataTypeStr=Bus: vehicle_attitude_bus
      settings: InheritFromInputs=off
  is_valid : Constant  Value=true  OutDataTypeStr=boolean
  vehicle_attitude : Outport  OutDataTypeStr=Bus: vehicle_attitude_bus  VectorParamsAs1DForOutWhenUnconnected=off
  wires:
  is_valid/1 -> Bus Creator/1
  timestamp_sample_imu/1 -> Bus Creator/2
  q/1 -> Bus Creator/3
  delta_q_reset/1 -> Bus Creator/4
  quat_reset_counter/1 -> Bus Creator/5
  Bus Creator/1 -> vehicle_attitude/1

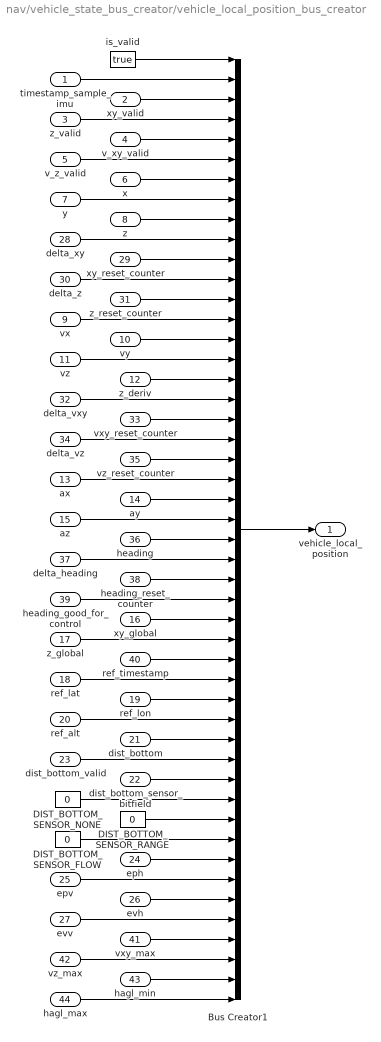
== system nav/vehicle_state_bus_creator/vehicle_local_position_bus_creator ==
  timestamp_sample_imu : Inport
  xy_valid : Inport  Port=2  OutDataTypeStr=boolean  PortDimensions=1
  z_valid : Inport  Port=3  OutDataTypeStr=boolean  PortDimensions=1
  v_xy_valid : Inport  Port=4  OutDataTypeStr=boolean  PortDimensions=1
  v_z_valid : Inport  Port=5  OutDataTypeStr=boolean  PortDimensions=1
  x : Inport  Port=6  OutDataTypeStr=single  PortDimensions=1
  y : Inport  Port=7  OutDataTypeStr=single  PortDimensions=1
  z : Inport  Port=8  OutDataTypeStr=single  PortDimensions=1
  vx : Inport  Port=9  OutDataTypeStr=single  PortDimensions=1
  vy : Inport  Port=10  OutDataTypeStr=single  PortDimensions=1
  vz : Inport  Port=11  OutDataTypeStr=single  PortDimensions=1
  z_deriv : Inport  Port=12  OutDataTypeStr=single  PortDimensions=1
  ax : Inport  Port=13  OutDataTypeStr=single  PortDimensions=1
  ay : Inport  Port=14  OutDataTypeStr=single  PortDimensions=1
  az : Inport  Port=15  OutDataTypeStr=single  PortDimensions=1
  xy_global : Inport  Port=16  OutDataTypeStr=boolean  PortDimensions=1
  z_global : Inport  Port=17  OutDataTypeStr=boolean  PortDimensions=1
  ref_lat : Inport  Port=18  OutDataTypeStr=double  PortDimensions=1
  ref_lon : Inport  Port=19  OutDataTypeStr=double  PortDimensions=1
  ref_alt : Inport  Port=20  OutDataTypeStr=single  PortDimensions=1
  dist_bottom : Inport  Port=21  OutDataTypeStr=single  PortDimensions=1
  dist_bottom_sensor_bitfield : Inport  Port=22  OutDataTypeStr=uint8  PortDimensions=1
  dist_bottom_valid : Inport  Port=23  OutDataTypeStr=boolean  PortDimensions=1
  eph : Inport  Port=24  OutDataTypeStr=single  PortDimensions=1
  epv : Inport  Port=25  OutDataTypeStr=single  PortDimensions=1
  evh : Inport  Port=26  OutDataTypeStr=single  PortDimensions=1
  evv : Inport  Port=27  OutDataTypeStr=single  PortDimensions=1
  delta_xy : Inport  Port=28  OutDataTypeStr=single  PortDimensions=2
  xy_reset_counter : Inport  Port=29  OutDataTypeStr=uint8  PortDimensions=1
  delta_z : Inport  Port=30  OutDataTypeStr=single  PortDimensions=1
  z_reset_counter : Inport  Port=31  OutDataTypeStr=uint8  PortDimensions=1
  delta_vxy : Inport  Port=32  OutDataTypeStr=single  PortDimensions=2
  vxy_reset_counter : Inport  Port=33  OutDataTypeStr=uint8  PortDimensions=1
  delta_vz : Inport  Port=34  OutDataTypeStr=single  PortDimensions=1
  vz_reset_counter : Inport  Port=35  OutDataTypeStr=uint8  PortDimensions=1
  heading : Inport  Port=36  OutDataTypeStr=single  PortDimensions=1
  delta_heading : Inport  Port=37  OutDataTypeStr=single  PortDimensions=1
  heading_reset_counter : Inport  Port=38  OutDataTypeStr=uint8  PortDimensions=1
  heading_good_for_control : Inport  Port=39  OutDataTypeStr=boolean  PortDimensions=1
  ref_timestamp : Inport  Port=40  OutDataTypeStr=double  PortDimensions=1
  vxy_max : Inport  Port=41  OutDataTypeStr=single  PortDimensions=1
  vz_max : Inport  Port=42  OutDataTypeStr=single  PortDimensions=1
  hagl_min : Inport  Port=43  OutDataTypeStr=single  PortDimensions=1
  hagl_max : Inport  Port=44  OutDataTypeStr=single  PortDimensions=1
  Bus Creator1 : BusCreator  Inputs=48  OutDataTypeStr=Bus: vehicle_local_position_bus
      settings: InheritFromInputs=off
  DIST_BOTTOM_SENSOR_FLOW : Constant  Value=0  OutDataTypeStr=uint8
  DIST_BOTTOM_SENSOR_NONE : Constant  Value=0  OutDataTypeStr=uint8
  DIST_BOTTOM_SENSOR_RANGE : Constant  Value=0  OutDataTypeStr=uint8
  is_valid : Constant  Value=true  OutDataTypeStr=boolean
  vehicle_local_position : Outport  OutDataTypeStr=Bus: vehicle_local_position_bus  VectorParamsAs1DForOutWhenUnconnected=off
  wires:
  is_valid/1 -> Bus Creator1/1
  xy_valid/1 -> Bus Creator1/3
  z_valid/1 -> Bus Creator1/4
  v_xy_valid/1 -> Bus Creator1/5
  v_z_valid/1 -> Bus Creator1/6
  x/1 -> Bus Creator1/7
  y/1 -> Bus Creator1/8
  z/1 -> Bus Creator1/9
  delta_xy/1 -> Bus Creator1/10
  xy_reset_counter/1 -> Bus Creator1/11
  delta_z/1 -> Bus Creator1/12
  z_reset_counter/1 -> Bus Creator1/13
  vx/1 -> Bus Creator1/14
  vy/1 -> Bus Creator1/15
  vz/1 -> Bus Creator1/16
  z_deriv/1 -> Bus Creator1/17
  delta_vxy/1 -> Bus Creator1/18
  vxy_reset_counter/1 -> Bus Creator1/19
  delta_vz/1 -> Bus Creator1/20
  vz_reset_counter/1 -> Bus Creator1/21
  ax/1 -> Bus Creator1/22
  ay/1 -> Bus Creator1/23
  az/1 -> Bus Creator1/24
  heading/1 -> Bus Creator1/25
  xy_global/1 -> Bus Creator1/29
  z_global/1 -> Bus Creator1/30
  ref_timestamp/1 -> Bus Creator1/31
  ref_lat/1 -> Bus Creator1/32
  ref_lon/1 -> Bus Creator1/33
  ref_alt/1 -> Bus Creator1/34
  dist_bottom/1 -> Bus Creator1/35
  dist_bottom_sensor_bitfield/1 -> Bus Creator1/37
  dist_bottom_valid/1 -> Bus Creator1/36
  eph/1 -> Bus Creator1/41
  epv/1 -> Bus Creator1/42
  evh/1 -> Bus Creator1/43
  evv/1 -> Bus Creator1/44
  vxy_max/1 -> Bus Creator1/45
  vz_max/1 -> Bus Creator1/46
  hagl_min/1 -> Bus Creator1/47
  hagl_max/1 -> Bus Creator1/48
  Bus Creator1/1 -> vehicle_local_position/1
  timestamp_sample_imu/1 -> Bus Creator1/2
  heading_good_for_control/1 -> Bus Creator1/28
  heading_reset_counter/1 -> Bus Creator1/27
  delta_heading/1 -> Bus Creator1/26
  DIST_BOTTOM_SENSOR_NONE/1 -> Bus Creator1/38
  DIST_BOTTOM_SENSOR_FLOW/1 -> Bus Creator1/40
  DIST_BOTTOM_SENSOR_RANGE/1 -> Bus Creator1/39

== matlab function nav/Actuator Model/cmd2deg ==
  data: act_limits input single; u input single; y output single
function y = fcn(act_limits,u)

y = u.*(act_limits*pi/180);

== matlab function nav/Actuator Model/limit control output ==
  data: u input single; y output single
function y = control_output_sat(u)

y = zeros(size(u),'single');
y(:) = min(max(u(:),-1),1);

end

== matlab function nav/vehicle_state_bus_creator/MATLAB Function ==
  data: acc_k input; gachi_dot output single size=2; Vk input
function gachi_dot = fcn(acc_k,Vk)
if Vk < single(0.5)
    Vk = single(0.5);
end

gachi_dot = [-acc_k(3);acc_k(2)]/Vk;

== matlab function nav/vehicle_state_bus_creator/acc transformation2 ==
  data: gachi_m input; acc_g input; acc_k output
function acc_k  = acc_transform(gachi_m,acc_g)

tf2 = [cos(gachi_m(1)) 0 -sin(gachi_m(1)); 0 1 0; sin(gachi_m(1)) 0 cos(gachi_m(1))];
tf3 = [cos(gachi_m(2)) sin(gachi_m(2)) 0; -sin(gachi_m(2)) cos(gachi_m(2)) 0; 0 0 1];

acc_k = tf2*tf3*(acc_g);

== matlab function nav/MATLAB Function8 ==
  data: gyro_raw input Bus: sensor_gyro_bus; gyro_m output; acc_raw input Bus: sensor_accel_bus; acc_m output; imu_filter input Bus: ifr_imu_filtered_bus; param input Bus: nav_parameterBus
function [gyro_m,acc_m] = fcn(gyro_raw,acc_raw,imu_filter,param)
pix_orientation = [param.pix_roll;param.pix_pitch;param.pix_yaw];

T1 = [1 0 0;0 cos(pix_orientation(1)) sin(pix_orientation(1));0 -sin(pix_orientation(1)) cos(pix_orientation(1))];
T2 = [cos(pix_orientation(2)) 0 -sin(pix_orientation(2));0 1 0;sin(pix_orientation(2)) 0 cos(pix_orientation(2))];
T3 = [cos(pix_orientation(3)) sin(pix_orientation(3)) 0;-sin(pix_orientation(3)) cos(pix_orientation(3)) 0;0 0 1];
T = T1*T2*T3;

if isequal(param.imu_filt.use_acc,single(1))
    acc_m = imu_filter.acc_filt;
else
    acc_m = T*[acc_raw.x;acc_raw.y;acc_raw.z];
end

if isequal(param.imu_filt.use_rte,single(1))
    gyro_m = imu_filter.rates_filt;
else
    gyro_m = T*[gyro_raw.x;gyro_raw.y;gyro_raw.z];
end

== matlab function nav/acc transformation4 ==
  data: acc_b input; euler input; acc_g output; navConsts parameter Bus: nav_constantsBus
function acc_g  = acc_transform(acc_b,euler,navConsts)

tf3 = [cos(-euler(3)) sin(-euler(3)) 0; -sin(-euler(3)) cos(-euler(3)) 0; 0 0 1];
tf2 = [cos(-euler(2)) 0 -sin(-euler(2)); 0 1 0; sin(-euler(2)) 0 cos(-euler(2))];
tf1 = [1 0 0; 0 cos(-euler(1)) sin(-euler(1)); 0 -sin(-euler(1)) cos(-euler(1))];

acc_g = tf3*tf2*tf1*(acc_b)+[0;0;navConsts.g];

== matlab function nav/barometer preprocessor ==
  settings: updateMethod=DISCRETE
  data: rawBaroData input Bus: sensor_baro_bus size=1; analysisParams output; height output; params input Bus: nav_parameterBus size=1; fixReference input boolean size=1; hil_on input; baro_rel output Bus: ifr_baro size=1; height_ref output; navConsts parameter
function [analysisParams,height,baro_rel,height_ref] = preprocessBaro(rawBaroData,params,fixReference,hil_on,navConsts)
persistent refHeight_dyn fixed
if params.dynRefHeight
    loopIdentifier = single(1);
    if isempty(refHeight_dyn)
        refHeight_dyn = single(navConsts.initialPositionLla(3));
        fixed=false;
        loopIdentifier = single(10);
    end
    if isempty(fixed)
        fixed=false;
        loopIdentifier = loopIdentifier+single(100);
    end
    
    baro_rel.isValid=(rawBaroData.is_valid && rawBaroData.pressure>500);
    height=computeHeightFromPressure(rawBaroData.pressure, navConsts);
    if ~fixed
        loopIdentifier = loopIdentifier+single(1000);
        baro_rel.height=single(0);
        if fixReference
            fixed=true;
        else
            if hil_on && navConsts.airStart %air start in simulation
            else
                refHeight_dyn = refHeight_dyn+params.biasSmoothingGain*(height-refHeight_dyn);
                loopIdentifier = loopIdentifier+single(10000);
            end
        end
    else
        baro_rel.height=height-refHeight_dyn;
        %baro.height=height;
    end
    height_ref = refHeight_dyn;
else
    loopIdentifier = single(0);
    refHeight_stat = params.referenceHeight;
    baro_rel.isValid=(rawBaroData.is_valid && rawBaroData.pressure>500);
    height=computeHeightFromPressure(rawBaroData.pressure, navConsts);
    if fixReference
        baro_rel.height=single(0);
    else
        baro_rel.height=height-refHeight_stat;
        %baro.height=height;
    end
    height_ref = refHeight_stat;
end
analysisParams = [navConsts.initialPositionLla(3),height,height_ref,loopIdentifier];
end

function height=computeHeightFromPressure(pressure, constants)
height=constants.referenceTemperature/constants.temperatureGradient*(1-(pressure/constants.referencePressure)^((constants.atmosphereKappa-1)/constants.atmosphereKappa));
end

== matlab function nav/delay compensation ==
  data: translation input single size=6; position output single size=3; attitude output single size=4; rotation input single size=4; delRot input single size=4; delPos input single size=3; delVel input single size=3; delAtt input single size=4; velocity output single size=3; navConsts parameter size=1
function [position, attitude, velocity] = fcn(translation,rotation,delRot,delPos,delVel,delAtt,navConsts)
    timeDelay=navConsts.filterDelay;
    
    geoToRef=quaternionProduct(delAtt, [delRot(1); -delRot(2:4)]);
    refToGeoMat=quatToMat(geoToRef)';
    position=delPos+timeDelay*delVel+refToGeoMat*translation(1:3)+0.5*timeDelay^2*[0; 0; navConsts.g];
    velocity=delVel+refToGeoMat*translation(4:6)+timeDelay*[0; 0; navConsts.g];
    attitude=quaternionProduct(geoToRef, rotation);
end

function prod=quaternionProduct(q, p)
    [q0, qVec, p0, pVec]=deal(q(1), q(2:4), p(1), p(2:4));
    prod=[q0*p0-qVec'*pVec; q0*pVec+p0*qVec+cross(qVec, pVec)];
end

function mat=quatToMat(quat)
    [q0, q1, q2, q3]=deal(quat(1), quat(2), quat(3), quat(4));
    mat=[1-2*(q2^2+q3^2), 2*(q1*q2+q3*q0), 2*(q1*q3-q2*q0); ...
         2*(q1*q2-q3*q0), 1-2*(q1^2+q3^2), 2*(q2*q3+q1*q0); ...
         2*(q1*q3+q2*q0), 2*(q2*q3-q1*q0), 1-2*(q1^2+q2^2)];
end
